simulink model "straight"  (R2015a)
settings: Solver=ode3  StartTime=0.0  StopTime=40  RelTol=1e-3
libraries: legoev3lib x4
settings Model: SimulationMode=external  ExtModeTrigDuration=2  Creator=USER  LastModifiedBy=USER
settings OptimizationCC: OptimizeModelRefInitCode=on  LifeSpan=1
settings DebuggingCC: UnderspecifiedInitializationDetection=Classic  MergeDetectMultiDrivingBlocksExec=none
settings HardwareCC: ProdLargestAtomicInteger=Long  ProdLargestAtomicFloat=Float  ProdEndianess=LittleEndian  ProdHWDeviceType=ARM Compatible->ARM 9
settings RTWCC: SystemTargetFile=realtime.tlc  GenerateMakefile=off  TemplateMakefile=realtime.tmf  Description=Run on Target Hardware  RTWVerbose=off
settings ERTTargetCC: CombineOutputUpdateFcns=off  ERTSrcFileBannerTemplate=realtime_code_template.cgt  ERTHdrFileBannerTemplate=realtime_code_template.cgt  ERTDataSrcFileTemplate=realtime_code_template.cgt  ERTDataHdrFileTemplate=realtime_code_template.cgt  ERTCustomFileTemplate=realtime_file_process.tlc

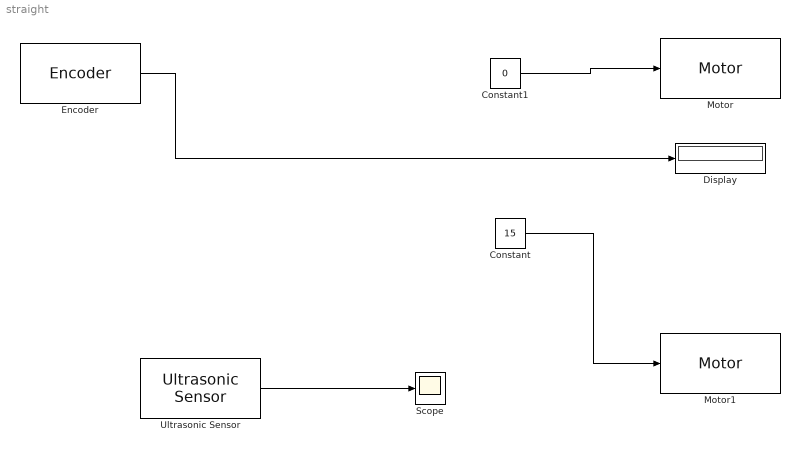
== system straight ==
  Constant : Constant  Value=15
  Constant1 : Constant  Value=0
  Display : Display
  Encoder : legoev3lib/Encoder  portNumber=B  opMode=No reset  sampleTime=0.1
  Motor : legoev3lib/Motor  sportNumber=B  sstopAction=Brake
  Motor1 : legoev3lib/Motor  sportNumber=A  sstopAction=Brake
  Scope : Scope
  Ultrasonic Sensor : legoev3lib/Ultrasonic Sensor  PortNumber=1  sampleTime=0.1
  wires:
  Constant/1 -> Motor1/1
  Encoder/1 -> Display/1
  Constant1/1 -> Motor/1
  Ultrasonic Sensor/1 -> Scope/1
